simulink model "sf_sawtooth1"  (R2020a)
settings: Solver=VariableStepAuto  StartTime=0.0  StopTime=10.0  RelTol=1e-3
settings Model: Creator=bzhan  LastModifiedBy=bzhan

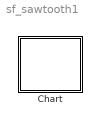
== system sf_sawtooth1 ==
  Chart : Stateflow chart  TreatAsAtomicUnit=on

== stateflow chart sf_sawtooth1/Chart ==
  settings: updateMethod=CONTINUOUS
  state A
    du: x_dot=1;
  (default) -> A : {x=0}
  A -> A : [x>=1]{x=0;}
  data: x local
  data x settings: updateMethod=SF_CONTINUOUS_TIME_DATA
